simulink model "Integral_Controller"  (R2022a)
settings: Solver=VariableStepAuto  StartTime=0.0  StopTime=10.0  RelTol=1e-3
undefined symbols (not defined in the file or in its folder): A_aug, B_aug, C_aug, D_aug, K, Ki, r
settings Model: Creator=yang  LastModifiedBy=yang

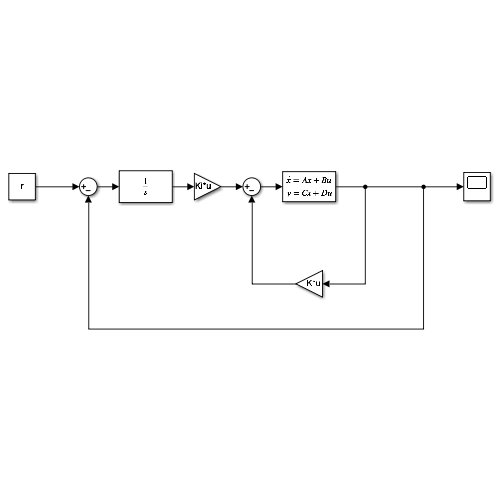
[thumbnail: Simulink's stored preview of the top-level diagram]
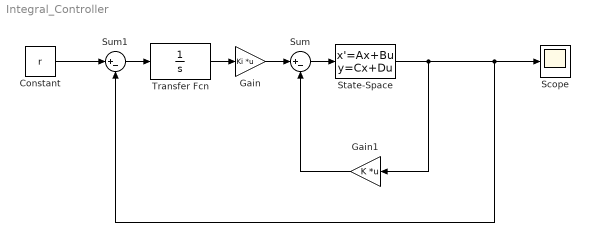
== system Integral_Controller ==
  Constant : Constant  Value=r
  Gain : Gain  Gain=Ki  Multiplication=Matrix(K*u)
  Gain1 : Gain  Gain=K  Multiplication=Matrix(K*u)
  Scope : Scope
  State-Space : StateSpace  A=A_aug  B=B_aug  C=C_aug  D=D_aug  InitialCondition=0
  Sum : Sum  Inputs=|+-
  Sum1 : Sum  Inputs=|+-
  Transfer Fcn : TransferFcn  Denominator=[1 0]
  wires:
  Transfer Fcn/1 -> Gain/1
  Gain/1 -> Sum/1
  Sum/1 -> State-Space/1
  Gain1/1 -> Sum/2
  Constant/1 -> Sum1/1
  Sum1/1 -> Transfer Fcn/1
  State-Space/1 -> Sum1/2, Scope/1, Gain1/1
